simulink subsystem "nonlinear_model"  (R2020b)
settings: Solver=VariableStepAuto  StartTime=0.0  StopTime=10.0  RelTol=1e-3
values from neighbouring files (symbols this model uses):
  Bp = 0.0024    [AAP5_setup.m]
  Br = 0.0024    [AAP5_setup.m]
  eta_g = 0.9    [AAP5_setup.m]
  eta_m = 0.69    [AAP5_setup.m]
  G = N4/N5 * N2/N3    (= 70)    [AAP5_setup.m]
  g = 9.81    [AAP5_setup.m]
  J = Jarm + Jrotor_eff    (= 0.00608016405667)    [AAP5_setup.m]
  Jp = mp*Lp^2/12    (= 0.00119873080146)    [AAP5_setup.m]
  kb = kt    (= 0.00768)    [AAP5_setup.m]
  kt = 7.68e-3    (= 0.00768)    [AAP5_setup.m]
  Lp = 0.33655    [AAP5_setup.m]
  lp = Lp/2    (= 0.168275)    [AAP5_setup.m]
  mp = 0.127    [AAP5_setup.m]
  r = 0.2159    [AAP5_setup.m]
  Ra = 2.6    [AAP5_setup.m]
settings Model: Creator=deniz  LastModifiedBy=deniz

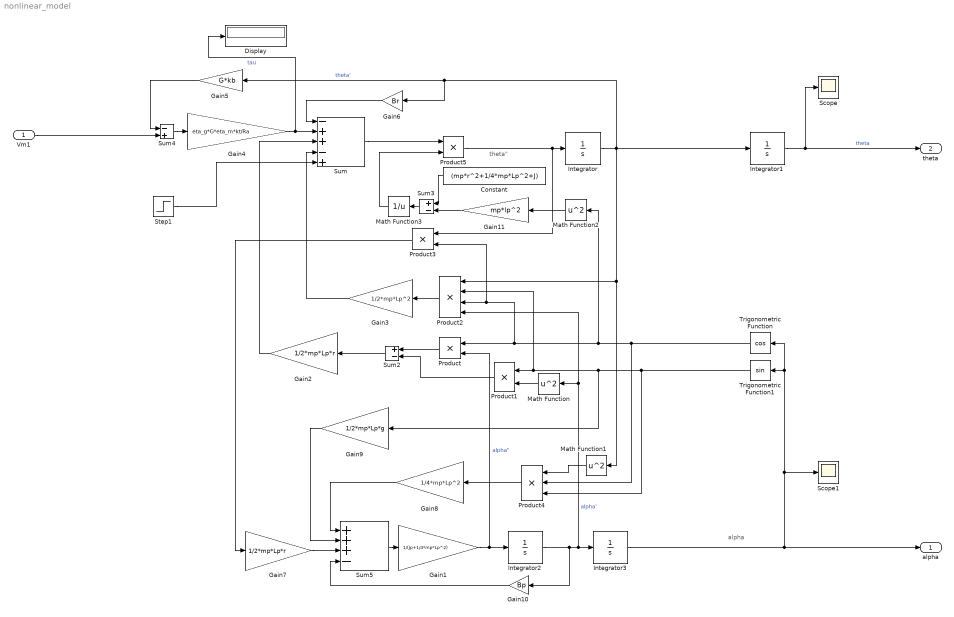
== system nonlinear_model ==
  note: theta"
  note: alpha
  Vm1 : Inport
  Constant : Constant  Value=(mp*r^2+1/4*mp*Lp^2+J)
  Display : Display
  Gain1 : Gain  Gain=1/(Jp+1/4*mp*Lp^2)
  Gain10 : Gain  Gain=Bp
  Gain11 : Gain  Gain=mp*lp^2
  Gain2 : Gain  Gain=1/2*mp*Lp*r
  Gain3 : Gain  Gain=1/2*mp*Lp^2
  Gain4 : Gain  Gain=eta_g*G*eta_m*kt/Ra
  Gain5 : Gain  Gain=G*kb
  Gain6 : Gain  Gain=Br
  Gain7 : Gain  Gain=1/2*mp*Lp*r
  Gain8 : Gain  Gain=1/4*mp*Lp^2
  Gain9 : Gain  Gain=1/2*mp*Lp*g
  Integrator{,1..3} (4 alike) : Integrator
  Math Function : Math  Operator=square  SignedPower=on  SaturateOnIntegerOverflow=on
  Math Function1 : Math  Operator=square  SignedPower=on  SaturateOnIntegerOverflow=on
  Math Function2 : Math  Operator=square  SignedPower=on  SaturateOnIntegerOverflow=on
  Math Function3 : Math  Operator=reciprocal  SignedPower=on  SaturateOnIntegerOverflow=on
  Product{,1,3,5} (4 alike) : Product  RndMeth=Zero
  Product2 : Product  Inputs=4  RndMeth=Zero
  Product4 : Product  Inputs=3  RndMeth=Zero
  Scope : Scope
  Scope1 : Scope
  Step1 : Step  Time=.1  After=0  SampleTime=0
  Sum : Sum  Inputs=-++-+
  Sum2 : Sum  Inputs=+-
  Sum3 : Sum  Inputs=+-
  Sum4 : Sum  Inputs=-+
  Sum5 : Sum  Inputs=+++-
  Trigonometric Function : Trigonometry  Operator=cos
  Trigonometric Function1 : Trigonometry
  alpha : Outport  VectorParamsAs1DForOutWhenUnconnected=off
  theta : Outport  Port=2  VectorParamsAs1DForOutWhenUnconnected=off
  wires:
  Product5/1 -> Integrator/1, Product3/1
  Product/1 -> Sum2/1
  Sum2/1 -> Gain2/1
  Sum/1 -> Product5/1
  Gain9/1 -> Sum5/2
  Gain10/1 -> Sum5/4
  Math Function2/1 -> Gain11/1
  Gain11/1 -> Sum3/2
  Constant/1 -> Sum3/1
  Sum3/1 -> Math Function3/1
  Math Function3/1 -> Product5/2
  Sum5/1 -> Gain1/1
  Gain2/1 -> Sum/3
  Gain7/1 -> Sum5/3
  Product3/1 -> Gain7/1
  Trigonometric Function1/1 -> Product1/1, Product2/2, Gain9/1, Product4/3
  Math Function/1 -> Product1/2
  Product1/1 -> Sum2/2
  Product4/1 -> Gain8/1
  Product2/1 -> Gain3/1
  Vm1/1 -> Sum4/2
  Gain5/1 -> Sum4/1
  Sum4/1 -> Gain4/1
  Gain4/1 -> Sum/2, Display/1  "tau"
  Gain6/1 -> Sum/1
  Gain3/1 -> Sum/4
  Gain8/1 -> Sum5/1
  Math Function1/1 -> Product4/1
  Integrator2/1 -> Product2/4, Math Function/1, Integrator3/1, Gain10/1  "alpha'"
  Gain1/1 -> Integrator2/1, Product/2  "alpha\""
  Trigonometric Function/1 -> Math Function2/1, Product/1, Product2/3, Product3/2, Product4/2
  Integrator/1 -> Gain5/1, Gain6/1, Integrator1/1, Product2/1, Math Function1/1  "theta'"
  Integrator1/1 -> Scope/1, theta/1  "theta"
  Step1/1 -> Sum/5
  Integrator3/1 -> alpha/1, Trigonometric Function1/1, Trigonometric Function/1, Scope1/1
